simulink model "testSiftOctave1"  (R2015a)
settings: Solver=ode45  StartTime=0.0  StopTime=20  RelTol=1e-3
InitFcn:
  | %% DSPBuilder Start
  | alt_dspbuilder_update_model(bdroot)
  | %% DSPBuilder End
libraries: allblocks_alteradspbuilder2 x2274
(part 15 of 26)

== system testSiftOctave1/sift_octave1/matching/compare_descriptor/get_distance ==
  hist_in1 : Inport
  hist_in2 : Inport  Port=2
  clken : Inport  Port=3
  BusSplitter : Subsystem
  BusSplitter1 : Subsystem
  Parallel Adder Subtractor : allblocks_alteradspbuilder2/Parallel Adder Subtractor  number_of_inputs=8  direction=+  use_pipeline=on  pipeline_display=3  phase_selection=1  use_ena=on  use_aclr=off  allowFloatingPointOverride=on  logOutputs=off  logFile=C:\Users\ASUS\Desktop\sift_fpga_final\Octave_2\tb_testSiftOctave1\testSiftOctave1_sift%5Foctave1_matching_compare%5Fdescriptor_get%5Fdistance_Parallel+Adder+Subtractor.fixedpointlog
  sub_GradOrian : Subsystem
  sub_GradOrian1 : Subsystem
  sub_GradOrian2 : Subsystem
  sub_GradOrian3 : Subsystem
  sub_GradOrian4 : Subsystem
  sub_GradOrian5 : Subsystem
  sub_GradOrian6 : Subsystem
  sub_GradOrian7 : Subsystem
  distance_out : Outport
  wires:
  hist_in2/1 -> [hist_in2]
  hist_in1/1 -> [hist_in1]
  [hist_in1] -> BusSplitter/1(data_in)
  [hist_in2] -> BusSplitter1/1(data_in)
  BusSplitter/1(bin1) -> [bin_11]
  BusSplitter/2(bin2) -> [bin_12]
  BusSplitter/3(bin3) -> [bin_13]
  BusSplitter/4(bin4) -> [bin_14]
  BusSplitter/5(bin5) -> [bin_15]
  BusSplitter/6(bin6) -> [bin_16]
  BusSplitter/7(bin7) -> [bin_17]
  BusSplitter/8(bin8) -> [bin_18]
  BusSplitter1/1(bin1) -> [bin_21]
  BusSplitter1/2(bin2) -> [bin_22]
  BusSplitter1/3(bin3) -> [bin_23]
  BusSplitter1/4(bin4) -> [bin_24]
  BusSplitter1/5(bin5) -> [bin_25]
  BusSplitter1/6(bin6) -> [bin_26]
  BusSplitter1/7(bin7) -> [bin_27]
  BusSplitter1/8(bin8) -> [bin_28]
  [bin_21] -> sub_GradOrian/2(bin2)
  [bin_11] -> sub_GradOrian/1(bin1)
  clken/1 -> [clken]
  [clken] -> sub_GradOrian/3(clken)
  sub_GradOrian/1(sub_bin) -> [sub_bin1]
  [bin_22] -> sub_GradOrian1/2(bin2)
  [bin_12] -> sub_GradOrian1/1(bin1)
  [clken] -> sub_GradOrian1/3(clken)
  sub_GradOrian1/1(sub_bin) -> [sub_bin2]
  [bin_23] -> sub_GradOrian2/2(bin2)
  [bin_13] -> sub_GradOrian2/1(bin1)
  [clken] -> sub_GradOrian2/3(clken)
  sub_GradOrian2/1(sub_bin) -> [sub_bin3]
  [bin_24] -> sub_GradOrian3/2(bin2)
  [bin_14] -> sub_GradOrian3/1(bin1)
  [clken] -> sub_GradOrian3/3(clken)
  sub_GradOrian3/1(sub_bin) -> [sub_bin4]
  [bin_25] -> sub_GradOrian4/2(bin2)
  [bin_15] -> sub_GradOrian4/1(bin1)
  [clken] -> sub_GradOrian4/3(clken)
  sub_GradOrian4/1(sub_bin) -> [sub_bin5]
  [bin_26] -> sub_GradOrian5/2(bin2)
  [bin_16] -> sub_GradOrian5/1(bin1)
  [clken] -> sub_GradOrian5/3(clken)
  sub_GradOrian5/1(sub_bin) -> [sub_bin6]
  [bin_27] -> sub_GradOrian6/2(bin2)
  [bin_17] -> sub_GradOrian6/1(bin1)
  [clken] -> sub_GradOrian6/3(clken)
  sub_GradOrian6/1(sub_bin) -> [sub_bin7]
  [bin_28] -> sub_GradOrian7/2(bin2)
  [bin_18] -> sub_GradOrian7/1(bin1)
  [clken] -> sub_GradOrian7/3(clken)
  sub_GradOrian7/1(sub_bin) -> [sub_bin8]
  [sub_bin1] -> Parallel Adder Subtractor/1
  [sub_bin2] -> Parallel Adder Subtractor/2
  [sub_bin3] -> Parallel Adder Subtractor/3
  [sub_bin4] -> Parallel Adder Subtractor/4
  [sub_bin5] -> Parallel Adder Subtractor/5
  [sub_bin6] -> Parallel Adder Subtractor/6
  [sub_bin7] -> Parallel Adder Subtractor/7
  [sub_bin8] -> Parallel Adder Subtractor/8
  [clken] -> Parallel Adder Subtractor/9
  Parallel Adder Subtractor/1 -> [distance_out]
  [distance_out] -> distance_out/1

== system testSiftOctave1/sift_octave1/matching/compare_descriptor/get_distance1 ==
  hist_in1 : Inport
  hist_in2 : Inport  Port=2
  clken : Inport  Port=3
  BusSplitter : Subsystem
  BusSplitter1 : Subsystem
  Parallel Adder Subtractor : allblocks_alteradspbuilder2/Parallel Adder Subtractor  number_of_inputs=8  direction=+  use_pipeline=on  pipeline_display=3  phase_selection=1  use_ena=on  use_aclr=off  allowFloatingPointOverride=on  logOutputs=off  logFile=C:\Users\ASUS\Desktop\sift_fpga_final\Octave_2\tb_testSiftOctave1\testSiftOctave1_sift%5Foctave1_matching_compare%5Fdescriptor_get%5Fdistance1_Parallel+Adder+Subtractor.fixedpointlog
  sub_GradOrian : Subsystem
  sub_GradOrian1 : Subsystem
  sub_GradOrian2 : Subsystem
  sub_GradOrian3 : Subsystem
  sub_GradOrian4 : Subsystem
  sub_GradOrian5 : Subsystem
  sub_GradOrian6 : Subsystem
  sub_GradOrian7 : Subsystem
  distance_out : Outport
  wires:
  hist_in2/1 -> [hist_in2]
  hist_in1/1 -> [hist_in1]
  [hist_in1] -> BusSplitter/1(data_in)
  [hist_in2] -> BusSplitter1/1(data_in)
  BusSplitter/1(bin1) -> [bin_11]
  BusSplitter/2(bin2) -> [bin_12]
  BusSplitter/3(bin3) -> [bin_13]
  BusSplitter/4(bin4) -> [bin_14]
  BusSplitter/5(bin5) -> [bin_15]
  BusSplitter/6(bin6) -> [bin_16]
  BusSplitter/7(bin7) -> [bin_17]
  BusSplitter/8(bin8) -> [bin_18]
  BusSplitter1/1(bin1) -> [bin_21]
  BusSplitter1/2(bin2) -> [bin_22]
  BusSplitter1/3(bin3) -> [bin_23]
  BusSplitter1/4(bin4) -> [bin_24]
  BusSplitter1/5(bin5) -> [bin_25]
  BusSplitter1/6(bin6) -> [bin_26]
  BusSplitter1/7(bin7) -> [bin_27]
  BusSplitter1/8(bin8) -> [bin_28]
  [bin_21] -> sub_GradOrian/2(bin2)
  [bin_11] -> sub_GradOrian/1(bin1)
  clken/1 -> [clken]
  [clken] -> sub_GradOrian/3(clken)
  sub_GradOrian/1(sub_bin) -> [sub_bin1]
  [bin_22] -> sub_GradOrian1/2(bin2)
  [bin_12] -> sub_GradOrian1/1(bin1)
  [clken] -> sub_GradOrian1/3(clken)
  sub_GradOrian1/1(sub_bin) -> [sub_bin2]
  [bin_23] -> sub_GradOrian2/2(bin2)
  [bin_13] -> sub_GradOrian2/1(bin1)
  [clken] -> sub_GradOrian2/3(clken)
  sub_GradOrian2/1(sub_bin) -> [sub_bin3]
  [bin_24] -> sub_GradOrian3/2(bin2)
  [bin_14] -> sub_GradOrian3/1(bin1)
  [clken] -> sub_GradOrian3/3(clken)
  sub_GradOrian3/1(sub_bin) -> [sub_bin4]
  [bin_25] -> sub_GradOrian4/2(bin2)
  [bin_15] -> sub_GradOrian4/1(bin1)
  [clken] -> sub_GradOrian4/3(clken)
  sub_GradOrian4/1(sub_bin) -> [sub_bin5]
  [bin_26] -> sub_GradOrian5/2(bin2)
  [bin_16] -> sub_GradOrian5/1(bin1)
  [clken] -> sub_GradOrian5/3(clken)
  sub_GradOrian5/1(sub_bin) -> [sub_bin6]
  [bin_27] -> sub_GradOrian6/2(bin2)
  [bin_17] -> sub_GradOrian6/1(bin1)
  [clken] -> sub_GradOrian6/3(clken)
  sub_GradOrian6/1(sub_bin) -> [sub_bin7]
  [bin_28] -> sub_GradOrian7/2(bin2)
  [bin_18] -> sub_GradOrian7/1(bin1)
  [clken] -> sub_GradOrian7/3(clken)
  sub_GradOrian7/1(sub_bin) -> [sub_bin8]
  [sub_bin1] -> Parallel Adder Subtractor/1
  [sub_bin2] -> Parallel Adder Subtractor/2
  [sub_bin3] -> Parallel Adder Subtractor/3
  [sub_bin4] -> Parallel Adder Subtractor/4
  [sub_bin5] -> Parallel Adder Subtractor/5
  [sub_bin6] -> Parallel Adder Subtractor/6
  [sub_bin7] -> Parallel Adder Subtractor/7
  [sub_bin8] -> Parallel Adder Subtractor/8
  [clken] -> Parallel Adder Subtractor/9
  Parallel Adder Subtractor/1 -> [distance_out]
  [distance_out] -> distance_out/1

== system testSiftOctave1/sift_octave1/matching/compare_descriptor/get_distance2 ==
  hist_in1 : Inport
  hist_in2 : Inport  Port=2
  clken : Inport  Port=3
  BusSplitter : Subsystem
  BusSplitter1 : Subsystem
  Parallel Adder Subtractor : allblocks_alteradspbuilder2/Parallel Adder Subtractor  number_of_inputs=8  direction=+  use_pipeline=on  pipeline_display=3  phase_selection=1  use_ena=on  use_aclr=off  allowFloatingPointOverride=on  logOutputs=off  logFile=C:\Users\ASUS\Desktop\sift_fpga_final\Octave_2\tb_testSiftOctave1\testSiftOctave1_sift%5Foctave1_matching_compare%5Fdescriptor_get%5Fdistance2_Parallel+Adder+Subtractor.fixedpointlog
  sub_GradOrian : Subsystem
  sub_GradOrian1 : Subsystem
  sub_GradOrian2 : Subsystem
  sub_GradOrian3 : Subsystem
  sub_GradOrian4 : Subsystem
  sub_GradOrian5 : Subsystem
  sub_GradOrian6 : Subsystem
  sub_GradOrian7 : Subsystem
  distance_out : Outport
  wires:
  hist_in2/1 -> [hist_in2]
  hist_in1/1 -> [hist_in1]
  [hist_in1] -> BusSplitter/1(data_in)
  [hist_in2] -> BusSplitter1/1(data_in)
  BusSplitter/1(bin1) -> [bin_11]
  BusSplitter/2(bin2) -> [bin_12]
  BusSplitter/3(bin3) -> [bin_13]
  BusSplitter/4(bin4) -> [bin_14]
  BusSplitter/5(bin5) -> [bin_15]
  BusSplitter/6(bin6) -> [bin_16]
  BusSplitter/7(bin7) -> [bin_17]
  BusSplitter/8(bin8) -> [bin_18]
  BusSplitter1/1(bin1) -> [bin_21]
  BusSplitter1/2(bin2) -> [bin_22]
  BusSplitter1/3(bin3) -> [bin_23]
  BusSplitter1/4(bin4) -> [bin_24]
  BusSplitter1/5(bin5) -> [bin_25]
  BusSplitter1/6(bin6) -> [bin_26]
  BusSplitter1/7(bin7) -> [bin_27]
  BusSplitter1/8(bin8) -> [bin_28]
  [bin_21] -> sub_GradOrian/2(bin2)
  [bin_11] -> sub_GradOrian/1(bin1)
  clken/1 -> [clken]
  [clken] -> sub_GradOrian/3(clken)
  sub_GradOrian/1(sub_bin) -> [sub_bin1]
  [bin_22] -> sub_GradOrian1/2(bin2)
  [bin_12] -> sub_GradOrian1/1(bin1)
  [clken] -> sub_GradOrian1/3(clken)
  sub_GradOrian1/1(sub_bin) -> [sub_bin2]
  [bin_23] -> sub_GradOrian2/2(bin2)
  [bin_13] -> sub_GradOrian2/1(bin1)
  [clken] -> sub_GradOrian2/3(clken)
  sub_GradOrian2/1(sub_bin) -> [sub_bin3]
  [bin_24] -> sub_GradOrian3/2(bin2)
  [bin_14] -> sub_GradOrian3/1(bin1)
  [clken] -> sub_GradOrian3/3(clken)
  sub_GradOrian3/1(sub_bin) -> [sub_bin4]
  [bin_25] -> sub_GradOrian4/2(bin2)
  [bin_15] -> sub_GradOrian4/1(bin1)
  [clken] -> sub_GradOrian4/3(clken)
  sub_GradOrian4/1(sub_bin) -> [sub_bin5]
  [bin_26] -> sub_GradOrian5/2(bin2)
  [bin_16] -> sub_GradOrian5/1(bin1)
  [clken] -> sub_GradOrian5/3(clken)
  sub_GradOrian5/1(sub_bin) -> [sub_bin6]
  [bin_27] -> sub_GradOrian6/2(bin2)
  [bin_17] -> sub_GradOrian6/1(bin1)
  [clken] -> sub_GradOrian6/3(clken)
  sub_GradOrian6/1(sub_bin) -> [sub_bin7]
  [bin_28] -> sub_GradOrian7/2(bin2)
  [bin_18] -> sub_GradOrian7/1(bin1)
  [clken] -> sub_GradOrian7/3(clken)
  sub_GradOrian7/1(sub_bin) -> [sub_bin8]
  [sub_bin1] -> Parallel Adder Subtractor/1
  [sub_bin2] -> Parallel Adder Subtractor/2
  [sub_bin3] -> Parallel Adder Subtractor/3
  [sub_bin4] -> Parallel Adder Subtractor/4
  [sub_bin5] -> Parallel Adder Subtractor/5
  [sub_bin6] -> Parallel Adder Subtractor/6
  [sub_bin7] -> Parallel Adder Subtractor/7
  [sub_bin8] -> Parallel Adder Subtractor/8
  [clken] -> Parallel Adder Subtractor/9
  Parallel Adder Subtractor/1 -> [distance_out]
  [distance_out] -> distance_out/1

== system testSiftOctave1/sift_octave1/matching/compare_descriptor/get_distance3 ==
  hist_in1 : Inport
  hist_in2 : Inport  Port=2
  clken : Inport  Port=3
  BusSplitter : Subsystem
  BusSplitter1 : Subsystem
  Parallel Adder Subtractor : allblocks_alteradspbuilder2/Parallel Adder Subtractor  number_of_inputs=8  direction=+  use_pipeline=on  pipeline_display=3  phase_selection=1  use_ena=on  use_aclr=off  allowFloatingPointOverride=on  logOutputs=off  logFile=C:\Users\ASUS\Desktop\sift_fpga_final\Octave_2\tb_testSiftOctave1\testSiftOctave1_sift%5Foctave1_matching_compare%5Fdescriptor_get%5Fdistance3_Parallel+Adder+Subtractor.fixedpointlog
  sub_GradOrian : Subsystem
  sub_GradOrian1 : Subsystem
  sub_GradOrian2 : Subsystem
  sub_GradOrian3 : Subsystem
  sub_GradOrian4 : Subsystem
  sub_GradOrian5 : Subsystem
  sub_GradOrian6 : Subsystem
  sub_GradOrian7 : Subsystem
  distance_out : Outport
  wires:
  hist_in2/1 -> [hist_in2]
  hist_in1/1 -> [hist_in1]
  [hist_in1] -> BusSplitter/1(data_in)
  [hist_in2] -> BusSplitter1/1(data_in)
  BusSplitter/1(bin1) -> [bin_11]
  BusSplitter/2(bin2) -> [bin_12]
  BusSplitter/3(bin3) -> [bin_13]
  BusSplitter/4(bin4) -> [bin_14]
  BusSplitter/5(bin5) -> [bin_15]
  BusSplitter/6(bin6) -> [bin_16]
  BusSplitter/7(bin7) -> [bin_17]
  BusSplitter/8(bin8) -> [bin_18]
  BusSplitter1/1(bin1) -> [bin_21]
  BusSplitter1/2(bin2) -> [bin_22]
  BusSplitter1/3(bin3) -> [bin_23]
  BusSplitter1/4(bin4) -> [bin_24]
  BusSplitter1/5(bin5) -> [bin_25]
  BusSplitter1/6(bin6) -> [bin_26]
  BusSplitter1/7(bin7) -> [bin_27]
  BusSplitter1/8(bin8) -> [bin_28]
  [bin_21] -> sub_GradOrian/2(bin2)
  [bin_11] -> sub_GradOrian/1(bin1)
  clken/1 -> [clken]
  [clken] -> sub_GradOrian/3(clken)
  sub_GradOrian/1(sub_bin) -> [sub_bin1]
  [bin_22] -> sub_GradOrian1/2(bin2)
  [bin_12] -> sub_GradOrian1/1(bin1)
  [clken] -> sub_GradOrian1/3(clken)
  sub_GradOrian1/1(sub_bin) -> [sub_bin2]
  [bin_23] -> sub_GradOrian2/2(bin2)
  [bin_13] -> sub_GradOrian2/1(bin1)
  [clken] -> sub_GradOrian2/3(clken)
  sub_GradOrian2/1(sub_bin) -> [sub_bin3]
  [bin_24] -> sub_GradOrian3/2(bin2)
  [bin_14] -> sub_GradOrian3/1(bin1)
  [clken] -> sub_GradOrian3/3(clken)
  sub_GradOrian3/1(sub_bin) -> [sub_bin4]
  [bin_25] -> sub_GradOrian4/2(bin2)
  [bin_15] -> sub_GradOrian4/1(bin1)
  [clken] -> sub_GradOrian4/3(clken)
  sub_GradOrian4/1(sub_bin) -> [sub_bin5]
  [bin_26] -> sub_GradOrian5/2(bin2)
  [bin_16] -> sub_GradOrian5/1(bin1)
  [clken] -> sub_GradOrian5/3(clken)
  sub_GradOrian5/1(sub_bin) -> [sub_bin6]
  [bin_27] -> sub_GradOrian6/2(bin2)
  [bin_17] -> sub_GradOrian6/1(bin1)
  [clken] -> sub_GradOrian6/3(clken)
  sub_GradOrian6/1(sub_bin) -> [sub_bin7]
  [bin_28] -> sub_GradOrian7/2(bin2)
  [bin_18] -> sub_GradOrian7/1(bin1)
  [clken] -> sub_GradOrian7/3(clken)
  sub_GradOrian7/1(sub_bin) -> [sub_bin8]
  [sub_bin1] -> Parallel Adder Subtractor/1
  [sub_bin2] -> Parallel Adder Subtractor/2
  [sub_bin3] -> Parallel Adder Subtractor/3
  [sub_bin4] -> Parallel Adder Subtractor/4
  [sub_bin5] -> Parallel Adder Subtractor/5
  [sub_bin6] -> Parallel Adder Subtractor/6
  [sub_bin7] -> Parallel Adder Subtractor/7
  [sub_bin8] -> Parallel Adder Subtractor/8
  [clken] -> Parallel Adder Subtractor/9
  Parallel Adder Subtractor/1 -> [distance_out]
  [distance_out] -> distance_out/1

== system testSiftOctave1/sift_octave1/matching/compare_descriptor/get_distance4 ==
  hist_in1 : Inport
  hist_in2 : Inport  Port=2
  clken : Inport  Port=3
  BusSplitter : Subsystem
  BusSplitter1 : Subsystem
  Parallel Adder Subtractor : allblocks_alteradspbuilder2/Parallel Adder Subtractor  number_of_inputs=8  direction=+  use_pipeline=on  pipeline_display=3  phase_selection=1  use_ena=on  use_aclr=off  allowFloatingPointOverride=on  logOutputs=off  logFile=C:\Users\ASUS\Desktop\sift_fpga_final\Octave_2\tb_testSiftOctave1\testSiftOctave1_sift%5Foctave1_matching_compare%5Fdescriptor_get%5Fdistance4_Parallel+Adder+Subtractor.fixedpointlog
  sub_GradOrian : Subsystem
  sub_GradOrian1 : Subsystem
  sub_GradOrian2 : Subsystem
  sub_GradOrian3 : Subsystem
  sub_GradOrian4 : Subsystem
  sub_GradOrian5 : Subsystem
  sub_GradOrian6 : Subsystem
  sub_GradOrian7 : Subsystem
  distance_out : Outport
  wires:
  hist_in2/1 -> [hist_in2]
  hist_in1/1 -> [hist_in1]
  [hist_in1] -> BusSplitter/1(data_in)
  [hist_in2] -> BusSplitter1/1(data_in)
  BusSplitter/1(bin1) -> [bin_11]
  BusSplitter/2(bin2) -> [bin_12]
  BusSplitter/3(bin3) -> [bin_13]
  BusSplitter/4(bin4) -> [bin_14]
  BusSplitter/5(bin5) -> [bin_15]
  BusSplitter/6(bin6) -> [bin_16]
  BusSplitter/7(bin7) -> [bin_17]
  BusSplitter/8(bin8) -> [bin_18]
  BusSplitter1/1(bin1) -> [bin_21]
  BusSplitter1/2(bin2) -> [bin_22]
  BusSplitter1/3(bin3) -> [bin_23]
  BusSplitter1/4(bin4) -> [bin_24]
  BusSplitter1/5(bin5) -> [bin_25]
  BusSplitter1/6(bin6) -> [bin_26]
  BusSplitter1/7(bin7) -> [bin_27]
  BusSplitter1/8(bin8) -> [bin_28]
  [bin_21] -> sub_GradOrian/2(bin2)
  [bin_11] -> sub_GradOrian/1(bin1)
  clken/1 -> [clken]
  [clken] -> sub_GradOrian/3(clken)
  sub_GradOrian/1(sub_bin) -> [sub_bin1]
  [bin_22] -> sub_GradOrian1/2(bin2)
  [bin_12] -> sub_GradOrian1/1(bin1)
  [clken] -> sub_GradOrian1/3(clken)
  sub_GradOrian1/1(sub_bin) -> [sub_bin2]
  [bin_23] -> sub_GradOrian2/2(bin2)
  [bin_13] -> sub_GradOrian2/1(bin1)
  [clken] -> sub_GradOrian2/3(clken)
  sub_GradOrian2/1(sub_bin) -> [sub_bin3]
  [bin_24] -> sub_GradOrian3/2(bin2)
  [bin_14] -> sub_GradOrian3/1(bin1)
  [clken] -> sub_GradOrian3/3(clken)
  sub_GradOrian3/1(sub_bin) -> [sub_bin4]
  [bin_25] -> sub_GradOrian4/2(bin2)
  [bin_15] -> sub_GradOrian4/1(bin1)
  [clken] -> sub_GradOrian4/3(clken)
  sub_GradOrian4/1(sub_bin) -> [sub_bin5]
  [bin_26] -> sub_GradOrian5/2(bin2)
  [bin_16] -> sub_GradOrian5/1(bin1)
  [clken] -> sub_GradOrian5/3(clken)
  sub_GradOrian5/1(sub_bin) -> [sub_bin6]
  [bin_27] -> sub_GradOrian6/2(bin2)
  [bin_17] -> sub_GradOrian6/1(bin1)
  [clken] -> sub_GradOrian6/3(clken)
  sub_GradOrian6/1(sub_bin) -> [sub_bin7]
  [bin_28] -> sub_GradOrian7/2(bin2)
  [bin_18] -> sub_GradOrian7/1(bin1)
  [clken] -> sub_GradOrian7/3(clken)
  sub_GradOrian7/1(sub_bin) -> [sub_bin8]
  [sub_bin1] -> Parallel Adder Subtractor/1
  [sub_bin2] -> Parallel Adder Subtractor/2
  [sub_bin3] -> Parallel Adder Subtractor/3
  [sub_bin4] -> Parallel Adder Subtractor/4
  [sub_bin5] -> Parallel Adder Subtractor/5
  [sub_bin6] -> Parallel Adder Subtractor/6
  [sub_bin7] -> Parallel Adder Subtractor/7
  [sub_bin8] -> Parallel Adder Subtractor/8
  [clken] -> Parallel Adder Subtractor/9
  Parallel Adder Subtractor/1 -> [distance_out]
  [distance_out] -> distance_out/1

== system testSiftOctave1/sift_octave1/matching/compare_descriptor/get_distance5 ==
  hist_in1 : Inport
  hist_in2 : Inport  Port=2
  clken : Inport  Port=3
  BusSplitter : Subsystem
  BusSplitter1 : Subsystem
  Parallel Adder Subtractor : allblocks_alteradspbuilder2/Parallel Adder Subtractor  number_of_inputs=8  direction=+  use_pipeline=on  pipeline_display=3  phase_selection=1  use_ena=on  use_aclr=off  allowFloatingPointOverride=on  logOutputs=off  logFile=C:\Users\ASUS\Desktop\sift_fpga_final\Octave_2\tb_testSiftOctave1\testSiftOctave1_sift%5Foctave1_matching_compare%5Fdescriptor_get%5Fdistance5_Parallel+Adder+Subtractor.fixedpointlog
  sub_GradOrian : Subsystem
  sub_GradOrian1 : Subsystem
  sub_GradOrian2 : Subsystem
  sub_GradOrian3 : Subsystem
  sub_GradOrian4 : Subsystem
  sub_GradOrian5 : Subsystem
  sub_GradOrian6 : Subsystem
  sub_GradOrian7 : Subsystem
  distance_out : Outport
  wires:
  hist_in2/1 -> [hist_in2]
  hist_in1/1 -> [hist_in1]
  [hist_in1] -> BusSplitter/1(data_in)
  [hist_in2] -> BusSplitter1/1(data_in)
  BusSplitter/1(bin1) -> [bin_11]
  BusSplitter/2(bin2) -> [bin_12]
  BusSplitter/3(bin3) -> [bin_13]
  BusSplitter/4(bin4) -> [bin_14]
  BusSplitter/5(bin5) -> [bin_15]
  BusSplitter/6(bin6) -> [bin_16]
  BusSplitter/7(bin7) -> [bin_17]
  BusSplitter/8(bin8) -> [bin_18]
  BusSplitter1/1(bin1) -> [bin_21]
  BusSplitter1/2(bin2) -> [bin_22]
  BusSplitter1/3(bin3) -> [bin_23]
  BusSplitter1/4(bin4) -> [bin_24]
  BusSplitter1/5(bin5) -> [bin_25]
  BusSplitter1/6(bin6) -> [bin_26]
  BusSplitter1/7(bin7) -> [bin_27]
  BusSplitter1/8(bin8) -> [bin_28]
  [bin_21] -> sub_GradOrian/2(bin2)
  [bin_11] -> sub_GradOrian/1(bin1)
  clken/1 -> [clken]
  [clken] -> sub_GradOrian/3(clken)
  sub_GradOrian/1(sub_bin) -> [sub_bin1]
  [bin_22] -> sub_GradOrian1/2(bin2)
  [bin_12] -> sub_GradOrian1/1(bin1)
  [clken] -> sub_GradOrian1/3(clken)
  sub_GradOrian1/1(sub_bin) -> [sub_bin2]
  [bin_23] -> sub_GradOrian2/2(bin2)
  [bin_13] -> sub_GradOrian2/1(bin1)
  [clken] -> sub_GradOrian2/3(clken)
  sub_GradOrian2/1(sub_bin) -> [sub_bin3]
  [bin_24] -> sub_GradOrian3/2(bin2)
  [bin_14] -> sub_GradOrian3/1(bin1)
  [clken] -> sub_GradOrian3/3(clken)
  sub_GradOrian3/1(sub_bin) -> [sub_bin4]
  [bin_25] -> sub_GradOrian4/2(bin2)
  [bin_15] -> sub_GradOrian4/1(bin1)
  [clken] -> sub_GradOrian4/3(clken)
  sub_GradOrian4/1(sub_bin) -> [sub_bin5]
  [bin_26] -> sub_GradOrian5/2(bin2)
  [bin_16] -> sub_GradOrian5/1(bin1)
  [clken] -> sub_GradOrian5/3(clken)
  sub_GradOrian5/1(sub_bin) -> [sub_bin6]
  [bin_27] -> sub_GradOrian6/2(bin2)
  [bin_17] -> sub_GradOrian6/1(bin1)
  [clken] -> sub_GradOrian6/3(clken)
  sub_GradOrian6/1(sub_bin) -> [sub_bin7]
  [bin_28] -> sub_GradOrian7/2(bin2)
  [bin_18] -> sub_GradOrian7/1(bin1)
  [clken] -> sub_GradOrian7/3(clken)
  sub_GradOrian7/1(sub_bin) -> [sub_bin8]
  [sub_bin1] -> Parallel Adder Subtractor/1
  [sub_bin2] -> Parallel Adder Subtractor/2
  [sub_bin3] -> Parallel Adder Subtractor/3
  [sub_bin4] -> Parallel Adder Subtractor/4
  [sub_bin5] -> Parallel Adder Subtractor/5
  [sub_bin6] -> Parallel Adder Subtractor/6
  [sub_bin7] -> Parallel Adder Subtractor/7
  [sub_bin8] -> Parallel Adder Subtractor/8
  [clken] -> Parallel Adder Subtractor/9
  Parallel Adder Subtractor/1 -> [distance_out]
  [distance_out] -> distance_out/1

== system testSiftOctave1/sift_octave1/matching/compare_descriptor/get_distance6 ==
  hist_in1 : Inport
  hist_in2 : Inport  Port=2
  clken : Inport  Port=3
  BusSplitter : Subsystem
  BusSplitter1 : Subsystem
  Parallel Adder Subtractor : allblocks_alteradspbuilder2/Parallel Adder Subtractor  number_of_inputs=8  direction=+  use_pipeline=on  pipeline_display=3  phase_selection=1  use_ena=on  use_aclr=off  allowFloatingPointOverride=on  logOutputs=off  logFile=C:\Users\ASUS\Desktop\sift_fpga_final\Octave_2\tb_testSiftOctave1\testSiftOctave1_sift%5Foctave1_matching_compare%5Fdescriptor_get%5Fdistance6_Parallel+Adder+Subtractor.fixedpointlog
  sub_GradOrian : Subsystem
  sub_GradOrian1 : Subsystem
  sub_GradOrian2 : Subsystem
  sub_GradOrian3 : Subsystem
  sub_GradOrian4 : Subsystem
  sub_GradOrian5 : Subsystem
  sub_GradOrian6 : Subsystem
  sub_GradOrian7 : Subsystem
  distance_out : Outport
  wires:
  hist_in2/1 -> [hist_in2]
  hist_in1/1 -> [hist_in1]
  [hist_in1] -> BusSplitter/1(data_in)
  [hist_in2] -> BusSplitter1/1(data_in)
  BusSplitter/1(bin1) -> [bin_11]
  BusSplitter/2(bin2) -> [bin_12]
  BusSplitter/3(bin3) -> [bin_13]
  BusSplitter/4(bin4) -> [bin_14]
  BusSplitter/5(bin5) -> [bin_15]
  BusSplitter/6(bin6) -> [bin_16]
  BusSplitter/7(bin7) -> [bin_17]
  BusSplitter/8(bin8) -> [bin_18]
  BusSplitter1/1(bin1) -> [bin_21]
  BusSplitter1/2(bin2) -> [bin_22]
  BusSplitter1/3(bin3) -> [bin_23]
  BusSplitter1/4(bin4) -> [bin_24]
  BusSplitter1/5(bin5) -> [bin_25]
  BusSplitter1/6(bin6) -> [bin_26]
  BusSplitter1/7(bin7) -> [bin_27]
  BusSplitter1/8(bin8) -> [bin_28]
  [bin_21] -> sub_GradOrian/2(bin2)
  [bin_11] -> sub_GradOrian/1(bin1)
  clken/1 -> [clken]
  [clken] -> sub_GradOrian/3(clken)
  sub_GradOrian/1(sub_bin) -> [sub_bin1]
  [bin_22] -> sub_GradOrian1/2(bin2)
  [bin_12] -> sub_GradOrian1/1(bin1)
  [clken] -> sub_GradOrian1/3(clken)
  sub_GradOrian1/1(sub_bin) -> [sub_bin2]
  [bin_23] -> sub_GradOrian2/2(bin2)
  [bin_13] -> sub_GradOrian2/1(bin1)
  [clken] -> sub_GradOrian2/3(clken)
  sub_GradOrian2/1(sub_bin) -> [sub_bin3]
  [bin_24] -> sub_GradOrian3/2(bin2)
  [bin_14] -> sub_GradOrian3/1(bin1)
  [clken] -> sub_GradOrian3/3(clken)
  sub_GradOrian3/1(sub_bin) -> [sub_bin4]
  [bin_25] -> sub_GradOrian4/2(bin2)
  [bin_15] -> sub_GradOrian4/1(bin1)
  [clken] -> sub_GradOrian4/3(clken)
  sub_GradOrian4/1(sub_bin) -> [sub_bin5]
  [bin_26] -> sub_GradOrian5/2(bin2)
  [bin_16] -> sub_GradOrian5/1(bin1)
  [clken] -> sub_GradOrian5/3(clken)
  sub_GradOrian5/1(sub_bin) -> [sub_bin6]
  [bin_27] -> sub_GradOrian6/2(bin2)
  [bin_17] -> sub_GradOrian6/1(bin1)
  [clken] -> sub_GradOrian6/3(clken)
  sub_GradOrian6/1(sub_bin) -> [sub_bin7]
  [bin_28] -> sub_GradOrian7/2(bin2)
  [bin_18] -> sub_GradOrian7/1(bin1)
  [clken] -> sub_GradOrian7/3(clken)
  sub_GradOrian7/1(sub_bin) -> [sub_bin8]
  [sub_bin1] -> Parallel Adder Subtractor/1
  [sub_bin2] -> Parallel Adder Subtractor/2
  [sub_bin3] -> Parallel Adder Subtractor/3
  [sub_bin4] -> Parallel Adder Subtractor/4
  [sub_bin5] -> Parallel Adder Subtractor/5
  [sub_bin6] -> Parallel Adder Subtractor/6
  [sub_bin7] -> Parallel Adder Subtractor/7
  [sub_bin8] -> Parallel Adder Subtractor/8
  [clken] -> Parallel Adder Subtractor/9
  Parallel Adder Subtractor/1 -> [distance_out]
  [distance_out] -> distance_out/1

== system testSiftOctave1/sift_octave1/matching/compare_descriptor/get_distance7 ==
  hist_in1 : Inport
  hist_in2 : Inport  Port=2
  clken : Inport  Port=3
  BusSplitter : Subsystem
  BusSplitter1 : Subsystem
  Parallel Adder Subtractor : allblocks_alteradspbuilder2/Parallel Adder Subtractor  number_of_inputs=8  direction=+  use_pipeline=on  pipeline_display=3  phase_selection=1  use_ena=on  use_aclr=off  allowFloatingPointOverride=on  logOutputs=off  logFile=C:\Users\ASUS\Desktop\sift_fpga_final\Octave_2\tb_testSiftOctave1\testSiftOctave1_sift%5Foctave1_matching_compare%5Fdescriptor_get%5Fdistance7_Parallel+Adder+Subtractor.fixedpointlog
  sub_GradOrian : Subsystem
  sub_GradOrian1 : Subsystem
  sub_GradOrian2 : Subsystem
  sub_GradOrian3 : Subsystem
  sub_GradOrian4 : Subsystem
  sub_GradOrian5 : Subsystem
  sub_GradOrian6 : Subsystem
  sub_GradOrian7 : Subsystem
  distance_out : Outport
  wires:
  hist_in2/1 -> [hist_in2]
  hist_in1/1 -> [hist_in1]
  [hist_in1] -> BusSplitter/1(data_in)
  [hist_in2] -> BusSplitter1/1(data_in)
  BusSplitter/1(bin1) -> [bin_11]
  BusSplitter/2(bin2) -> [bin_12]
  BusSplitter/3(bin3) -> [bin_13]
  BusSplitter/4(bin4) -> [bin_14]
  BusSplitter/5(bin5) -> [bin_15]
  BusSplitter/6(bin6) -> [bin_16]
  BusSplitter/7(bin7) -> [bin_17]
  BusSplitter/8(bin8) -> [bin_18]
  BusSplitter1/1(bin1) -> [bin_21]
  BusSplitter1/2(bin2) -> [bin_22]
  BusSplitter1/3(bin3) -> [bin_23]
  BusSplitter1/4(bin4) -> [bin_24]
  BusSplitter1/5(bin5) -> [bin_25]
  BusSplitter1/6(bin6) -> [bin_26]
  BusSplitter1/7(bin7) -> [bin_27]
  BusSplitter1/8(bin8) -> [bin_28]
  [bin_21] -> sub_GradOrian/2(bin2)
  [bin_11] -> sub_GradOrian/1(bin1)
  clken/1 -> [clken]
  [clken] -> sub_GradOrian/3(clken)
  sub_GradOrian/1(sub_bin) -> [sub_bin1]
  [bin_22] -> sub_GradOrian1/2(bin2)
  [bin_12] -> sub_GradOrian1/1(bin1)
  [clken] -> sub_GradOrian1/3(clken)
  sub_GradOrian1/1(sub_bin) -> [sub_bin2]
  [bin_23] -> sub_GradOrian2/2(bin2)
  [bin_13] -> sub_GradOrian2/1(bin1)
  [clken] -> sub_GradOrian2/3(clken)
  sub_GradOrian2/1(sub_bin) -> [sub_bin3]
  [bin_24] -> sub_GradOrian3/2(bin2)
  [bin_14] -> sub_GradOrian3/1(bin1)
  [clken] -> sub_GradOrian3/3(clken)
  sub_GradOrian3/1(sub_bin) -> [sub_bin4]
  [bin_25] -> sub_GradOrian4/2(bin2)
  [bin_15] -> sub_GradOrian4/1(bin1)
  [clken] -> sub_GradOrian4/3(clken)
  sub_GradOrian4/1(sub_bin) -> [sub_bin5]
  [bin_26] -> sub_GradOrian5/2(bin2)
  [bin_16] -> sub_GradOrian5/1(bin1)
  [clken] -> sub_GradOrian5/3(clken)
  sub_GradOrian5/1(sub_bin) -> [sub_bin6]
  [bin_27] -> sub_GradOrian6/2(bin2)
  [bin_17] -> sub_GradOrian6/1(bin1)
  [clken] -> sub_GradOrian6/3(clken)
  sub_GradOrian6/1(sub_bin) -> [sub_bin7]
  [bin_28] -> sub_GradOrian7/2(bin2)
  [bin_18] -> sub_GradOrian7/1(bin1)
  [clken] -> sub_GradOrian7/3(clken)
  sub_GradOrian7/1(sub_bin) -> [sub_bin8]
  [sub_bin1] -> Parallel Adder Subtractor/1
  [sub_bin2] -> Parallel Adder Subtractor/2
  [sub_bin3] -> Parallel Adder Subtractor/3
  [sub_bin4] -> Parallel Adder Subtractor/4
  [sub_bin5] -> Parallel Adder Subtractor/5
  [sub_bin6] -> Parallel Adder Subtractor/6
  [sub_bin7] -> Parallel Adder Subtractor/7
  [sub_bin8] -> Parallel Adder Subtractor/8
  [clken] -> Parallel Adder Subtractor/9
  Parallel Adder Subtractor/1 -> [distance_out]
  [distance_out] -> distance_out/1

== system testSiftOctave1/sift_octave1/matching/compare_descriptor/get_distance8 ==
  hist_in1 : Inport
  hist_in2 : Inport  Port=2
  clken : Inport  Port=3
  BusSplitter : Subsystem
  BusSplitter1 : Subsystem
  Parallel Adder Subtractor : allblocks_alteradspbuilder2/Parallel Adder Subtractor  number_of_inputs=8  direction=+  use_pipeline=on  pipeline_display=3  phase_selection=1  use_ena=on  use_aclr=off  allowFloatingPointOverride=on  logOutputs=off  logFile=C:\Users\ASUS\Desktop\sift_fpga_final\Octave_2\tb_testSiftOctave1\testSiftOctave1_sift%5Foctave1_matching_compare%5Fdescriptor_get%5Fdistance8_Parallel+Adder+Subtractor.fixedpointlog
  sub_GradOrian : Subsystem
  sub_GradOrian1 : Subsystem
  sub_GradOrian2 : Subsystem
  sub_GradOrian3 : Subsystem
  sub_GradOrian4 : Subsystem
  sub_GradOrian5 : Subsystem
  sub_GradOrian6 : Subsystem
  sub_GradOrian7 : Subsystem
  distance_out : Outport
  wires:
  hist_in2/1 -> [hist_in2]
  hist_in1/1 -> [hist_in1]
  [hist_in1] -> BusSplitter/1(data_in)
  [hist_in2] -> BusSplitter1/1(data_in)
  BusSplitter/1(bin1) -> [bin_11]
  BusSplitter/2(bin2) -> [bin_12]
  BusSplitter/3(bin3) -> [bin_13]
  BusSplitter/4(bin4) -> [bin_14]
  BusSplitter/5(bin5) -> [bin_15]
  BusSplitter/6(bin6) -> [bin_16]
  BusSplitter/7(bin7) -> [bin_17]
  BusSplitter/8(bin8) -> [bin_18]
  BusSplitter1/1(bin1) -> [bin_21]
  BusSplitter1/2(bin2) -> [bin_22]
  BusSplitter1/3(bin3) -> [bin_23]
  BusSplitter1/4(bin4) -> [bin_24]
  BusSplitter1/5(bin5) -> [bin_25]
  BusSplitter1/6(bin6) -> [bin_26]
  BusSplitter1/7(bin7) -> [bin_27]
  BusSplitter1/8(bin8) -> [bin_28]
  [bin_21] -> sub_GradOrian/2(bin2)
  [bin_11] -> sub_GradOrian/1(bin1)
  clken/1 -> [clken]
  [clken] -> sub_GradOrian/3(clken)
  sub_GradOrian/1(sub_bin) -> [sub_bin1]
  [bin_22] -> sub_GradOrian1/2(bin2)
  [bin_12] -> sub_GradOrian1/1(bin1)
  [clken] -> sub_GradOrian1/3(clken)
  sub_GradOrian1/1(sub_bin) -> [sub_bin2]
  [bin_23] -> sub_GradOrian2/2(bin2)
  [bin_13] -> sub_GradOrian2/1(bin1)
  [clken] -> sub_GradOrian2/3(clken)
  sub_GradOrian2/1(sub_bin) -> [sub_bin3]
  [bin_24] -> sub_GradOrian3/2(bin2)
  [bin_14] -> sub_GradOrian3/1(bin1)
  [clken] -> sub_GradOrian3/3(clken)
  sub_GradOrian3/1(sub_bin) -> [sub_bin4]
  [bin_25] -> sub_GradOrian4/2(bin2)
  [bin_15] -> sub_GradOrian4/1(bin1)
  [clken] -> sub_GradOrian4/3(clken)
  sub_GradOrian4/1(sub_bin) -> [sub_bin5]
  [bin_26] -> sub_GradOrian5/2(bin2)
  [bin_16] -> sub_GradOrian5/1(bin1)
  [clken] -> sub_GradOrian5/3(clken)
  sub_GradOrian5/1(sub_bin) -> [sub_bin6]
  [bin_27] -> sub_GradOrian6/2(bin2)
  [bin_17] -> sub_GradOrian6/1(bin1)
  [clken] -> sub_GradOrian6/3(clken)
  sub_GradOrian6/1(sub_bin) -> [sub_bin7]
  [bin_28] -> sub_GradOrian7/2(bin2)
  [bin_18] -> sub_GradOrian7/1(bin1)
  [clken] -> sub_GradOrian7/3(clken)
  sub_GradOrian7/1(sub_bin) -> [sub_bin8]
  [sub_bin1] -> Parallel Adder Subtractor/1
  [sub_bin2] -> Parallel Adder Subtractor/2
  [sub_bin3] -> Parallel Adder Subtractor/3
  [sub_bin4] -> Parallel Adder Subtractor/4
  [sub_bin5] -> Parallel Adder Subtractor/5
  [sub_bin6] -> Parallel Adder Subtractor/6
  [sub_bin7] -> Parallel Adder Subtractor/7
  [sub_bin8] -> Parallel Adder Subtractor/8
  [clken] -> Parallel Adder Subtractor/9
  Parallel Adder Subtractor/1 -> [distance_out]
  [distance_out] -> distance_out/1

== system testSiftOctave1/sift_octave1/matching/compare_descriptor/isDescriptor ==
  descriptor1 : Inport
  descriptor2 : Inport  Port=2
  addr1_in : Inport  Port=3
  addr2_in : Inport  Port=4
  Comparator : allblocks_alteradspbuilder2/Comparator  direction=a == b  pipeline_display=0  allowFloatingPointOverride=on  logOutputs=off  logFile=C:\Users\ASUS\Desktop\sift_fpga_final\Octave_2\tb_testSiftOctave1\testSiftOctave1_sift%5Foctave1_matching_compare%5Fdescriptor_isDescriptor_Comparator.fixedpointlog
  Comparator1 : allblocks_alteradspbuilder2/Comparator  direction=a == b  pipeline_display=0  allowFloatingPointOverride=on  logOutputs=off  logFile=C:\Users\ASUS\Desktop\sift_fpga_final\Octave_2\tb_testSiftOctave1\testSiftOctave1_sift%5Foctave1_matching_compare%5Fdescriptor_isDescriptor_Comparator1.fixedpointlog
  Comparator2 : allblocks_alteradspbuilder2/Comparator  direction=a == b  pipeline_display=0  allowFloatingPointOverride=on  logOutputs=off  logFile=C:\Users\ASUS\Desktop\sift_fpga_final\Octave_2\tb_testSiftOctave1\testSiftOctave1_sift%5Foctave1_matching_compare%5Fdescriptor_isDescriptor_Comparator2.fixedpointlog
  Comparator3 : allblocks_alteradspbuilder2/Comparator  direction=a == b  pipeline_display=0  allowFloatingPointOverride=on  logOutputs=off  logFile=C:\Users\ASUS\Desktop\sift_fpga_final\Octave_2\tb_testSiftOctave1\testSiftOctave1_sift%5Foctave1_matching_compare%5Fdescriptor_isDescriptor_Comparator3.fixedpointlog
  Constant : allblocks_alteradspbuilder2/Constant  mask_cst=1998  BusType=Signed Integer  bwl=1172  bwr=0  roundMode=Truncate  satMode=Wrap  SpecifyClock=off  allowFloatingPointOverride=on  logOutputs=off  logFile=C:\Users\ASUS\Desktop\sift_fpga_final\Octave_2\tb_testSiftOctave1\testSiftOctave1_sift%5Foctave1_matching_compare%5Fdescriptor_isDescriptor_Constant.fixedpointlog
  Constant1 : allblocks_alteradspbuilder2/Constant  mask_cst=1998  BusType=Signed Integer  bwl=1172  bwr=0  roundMode=Truncate  satMode=Wrap  SpecifyClock=off  allowFloatingPointOverride=on  logOutputs=off  logFile=C:\Users\ASUS\Desktop\sift_fpga_final\Octave_2\tb_testSiftOctave1\testSiftOctave1_sift%5Foctave1_matching_compare%5Fdescriptor_isDescriptor_Constant1.fixedpointlog
  Constant2 : allblocks_alteradspbuilder2/Constant  mask_cst=1  BusType=Single Bit  bwl=1172  bwr=0  roundMode=Truncate  satMode=Wrap  SpecifyClock=off  allowFloatingPointOverride=on  logOutputs=off  logFile=C:\Users\ASUS\Desktop\sift_fpga_final\Octave_2\tb_testSiftOctave1\testSiftOctave1_sift%5Foctave1_matching_compare%5Fdescriptor_isDescriptor_Constant2.fixedpointlog
  Constant3 : allblocks_alteradspbuilder2/Constant  mask_cst=1  BusType=Single Bit  bwl=1172  bwr=0  roundMode=Truncate  satMode=Wrap  SpecifyClock=off  allowFloatingPointOverride=on  logOutputs=off  logFile=C:\Users\ASUS\Desktop\sift_fpga_final\Octave_2\tb_testSiftOctave1\testSiftOctave1_sift%5Foctave1_matching_compare%5Fdescriptor_isDescriptor_Constant3.fixedpointlog
  Constant4 : allblocks_alteradspbuilder2/Constant  mask_cst=0  BusType=Unsigned Integer  bwl=10  bwr=0  roundMode=Truncate  satMode=Wrap  SpecifyClock=off  allowFloatingPointOverride=on  logOutputs=off  logFile=C:\Users\ASUS\Desktop\sift_fpga_final\Octave_2\tb_testSiftOctave1\testSiftOctave1_sift%5Foctave1_matching_compare%5Fdescriptor_isDescriptor_Constant4.fixedpointlog
  Constant5 : allblocks_alteradspbuilder2/Constant  mask_cst=0  BusType=Unsigned Integer  bwl=10  bwr=0  roundMode=Truncate  satMode=Wrap  SpecifyClock=off  allowFloatingPointOverride=on  logOutputs=off  logFile=C:\Users\ASUS\Desktop\sift_fpga_final\Octave_2\tb_testSiftOctave1\testSiftOctave1_sift%5Foctave1_matching_compare%5Fdescriptor_isDescriptor_Constant5.fixedpointlog
  Constant6 : allblocks_alteradspbuilder2/Constant  mask_cst=1  BusType=Single Bit  bwl=1172  bwr=0  roundMode=Truncate  satMode=Wrap  SpecifyClock=off  allowFloatingPointOverride=on  logOutputs=off  logFile=C:\Users\ASUS\Desktop\sift_fpga_final\Octave_2\tb_testSiftOctave1\testSiftOctave1_sift%5Foctave1_matching_compare%5Fdescriptor_isDescriptor_Constant6.fixedpointlog
  Constant7 : allblocks_alteradspbuilder2/Constant  mask_cst=0  BusType=Single Bit  bwl=1172  bwr=0  roundMode=Truncate  satMode=Wrap  SpecifyClock=off  allowFloatingPointOverride=on  logOutputs=off  logFile=C:\Users\ASUS\Desktop\sift_fpga_final\Octave_2\tb_testSiftOctave1\testSiftOctave1_sift%5Foctave1_matching_compare%5Fdescriptor_isDescriptor_Constant7.fixedpointlog
  Flipflop : allblocks_alteradspbuilder2/Flipflop  mode=DFFE  BusType=Single Bit  bwl=10  bwr=2  pipeline_display=1
  Flipflop1 : allblocks_alteradspbuilder2/Flipflop  mode=DFFE  BusType=Unsigned Integer  bwl=10  bwr=2  pipeline_display=1
  Logical Bit Operator : allblocks_alteradspbuilder2/Logical Bit Operator  LogicalOperator=OR  user_inputs=2  pipeline_display=0
  Multiplexer : allblocks_alteradspbuilder2/Multiplexer  numInputs=2  pipeline=0  oneHot=off  pipeline_display=0  use_ena=off  use_aclr=off  allowFloatingPointOverride=on  logOutputs=off  logFile=C:\Users\ASUS\Desktop\sift_fpga_final\Octave_2\tb_testSiftOctave1\testSiftOctave1_sift%5Foctave1_matching_compare%5Fdescriptor_isDescriptor_Multiplexer.fixedpointlog
  isDescriptor : Outport
  wires:
  Constant3/1 -> Flipflop1/1
  Comparator2/1 -> Flipflop/3, Flipflop/4
  [addr2_in] -> Comparator3/1
  Comparator3/1 -> Flipflop1/4, Flipflop1/3
  Constant5/1 -> Comparator3/2
  [addr1_in] -> Comparator2/1
  Constant4/1 -> Comparator2/2
  Flipflop1/1 -> Logical Bit Operator/2
  descriptor1/1 -> [descriptor1]
  addr1_in/1 -> [addr1_in]
  descriptor2/1 -> [descriptor2]
  addr2_in/1 -> [addr2_in]
  Flipflop/1 -> Logical Bit Operator/1
  Constant1/1 -> Comparator1/2
  [descriptor1] -> Comparator/1
  Comparator1/1 -> Flipflop1/2
  Comparator/1 -> Flipflop/2
  [descriptor2] -> Comparator1/1
  Constant/1 -> Comparator/2
  Constant2/1 -> Flipflop/1
  Logical Bit Operator/1 -> Multiplexer/1
  Constant6/1 -> Multiplexer/2
  Constant7/1 -> Multiplexer/3
  Multiplexer/1 -> isDescriptor/1

== system testSiftOctave1/sift_octave1/matching/draw_keypoint_match/counter ==
  valid_in : Inport
  eof_in : Inport  Port=2
  Comparator : allblocks_alteradspbuilder2/Comparator  direction=a == b  pipeline_display=0  allowFloatingPointOverride=on  logOutputs=off  logFile=C:\Users\ASUS\Desktop\sift_fpga_final\Octave_2\tb_testSiftOctave1\testSiftOctave1_sift%5Foctave1_matching_draw%5Fkeypoint%5Fmatch_counter_Comparator.fixedpointlog
  Constant : allblocks_alteradspbuilder2/Constant  mask_cst=639  BusType=Unsigned Integer  bwl=10  bwr=0  roundMode=Truncate  satMode=Wrap  SpecifyClock=off  allowFloatingPointOverride=on  logOutputs=off  logFile=C:\Users\ASUS\Desktop\sift_fpga_final\Octave_2\tb_testSiftOctave1\testSiftOctave1_sift%5Foctave1_matching_draw%5Fkeypoint%5Fmatch_counter_Constant.fixedpointlog
  Counter : allblocks_alteradspbuilder2/Counter  BusType=Unsigned Integer  bwl=10  bwr=0  use_modulo=on  modulo=640  SpecifyClock=off  direction=Increment  use_sload=off  use_sset=off  svalue=0  use_clk_ena=off  use_ena=on  use_sclr=on  pipeline_display=1
  Counter1 : allblocks_alteradspbuilder2/Counter  BusType=Unsigned Integer  bwl=10  bwr=0  use_modulo=on  modulo=480  SpecifyClock=off  direction=Increment  use_sload=off  use_sset=off  svalue=0  use_clk_ena=off  use_ena=on  use_sclr=on  pipeline_display=1
  Logical Bit Operator : allblocks_alteradspbuilder2/Logical Bit Operator  LogicalOperator=AND  user_inputs=2  pipeline_display=0
  col_out : Outport
  row_out : Outport  Port=2
  wires:
  [eof_in] -> Counter1/2
  Logical Bit Operator/1 -> Counter1/1
  [counter_col] -> Comparator/1
  eof_in/1 -> [eof_in]
  Constant/1 -> Comparator/2
  Comparator/1 -> Logical Bit Operator/2
  valid_in/1 -> [valid_in]
  Counter1/1 -> [counter_row]
  Counter/1 -> [counter_col]
  [valid_in] -> Logical Bit Operator/1, Counter/1
  [counter_row] -> row_out/1
  [counter_col] -> col_out/1
  [eof_in] -> Counter/2
